simulink library "EarthAndTargetPointing"  (R2014b)
settings: Solver=ode45  StartTime=0.0  StopTime=10.0  RelTol=1e-3
undefined symbols (not defined in the file or in its folder): ConfParam
libraries: AdvancedMux x2, Normalization x2, AdvancedDemux x1, ComputeNorm3D x1, EarthPointing x1, ScalarProduct3D x1, TargetPointing x1
settings Model: Creator=Hp  LastModifiedBy=Hp

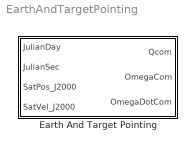
== system EarthAndTargetPointing ==
  Earth And Target Pointing : Subsystem

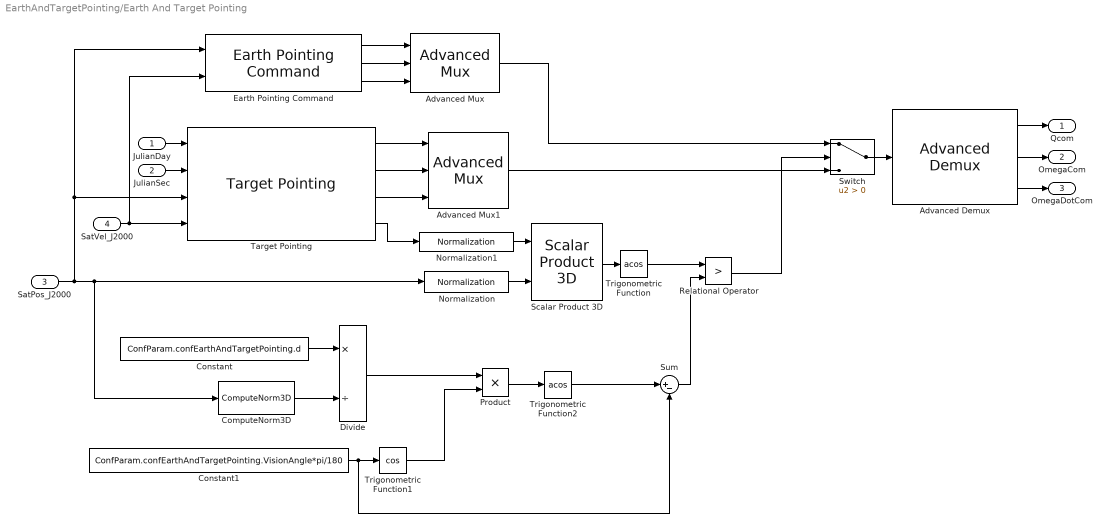
== system EarthAndTargetPointing/Earth And Target Pointing ==
  JulianDay : Inport
  JulianSec : Inport  Port=2
  SatPos_J2000 : Inport  Port=3
  SatVel_J2000 : Inport  Port=4
  Advanced Demux : AdvancedDemux/Advanced Demux
  Advanced Mux : AdvancedMux/Advanced Mux
  Advanced Mux1 : AdvancedMux/Advanced Mux
  ComputeNorm3D : ComputeNorm3D/ComputeNorm3D
  Constant : Constant  Value=ConfParam.confEarthAndTargetPointing.d
  Constant1 : Constant  Value=ConfParam.confEarthAndTargetPointing.VisionAngle*pi/180
  Divide : Product  Inputs=*/
  "Earth Pointing Command " : EarthPointing/Earth Pointing Command
  Normalization : Normalization/Normalization
  Normalization1 : Normalization/Normalization
  Product : Product
  Relational Operator : RelationalOperator  Operator=>  OutDataTypeStr=boolean
  Scalar Product 3D : ScalarProduct3D/Scalar Product 3D
  Sum : Sum  Inputs=|+-
  Switch : Switch  Criteria=u2 > Threshold
  Target Pointing : TargetPointing/Target Pointing
  Trigonometric Function : Trigonometry  Operator=acos
  Trigonometric Function1 : Trigonometry  Operator=cos
  Trigonometric Function2 : Trigonometry  Operator=acos
  Qcom : Outport
  OmegaCom : Outport  Port=2
  OmegaDotCom : Outport  Port=3
  wires:
  JulianSec/1 -> Target Pointing/2
  Normalization1/1 -> Scalar Product 3D/1
  Normalization/1 -> Scalar Product 3D/2
  SatPos_J2000/1 -> Target Pointing/3, "Earth Pointing Command "/1, ComputeNorm3D/1, Normalization/1
  JulianDay/1 -> Target Pointing/1
  Trigonometric Function/1 -> Relational Operator/1
  Scalar Product 3D/1 -> Trigonometric Function/1
  SatVel_J2000/1 -> Target Pointing/4, "Earth Pointing Command "/2
  Target Pointing/4 -> Normalization1/1
  "Earth Pointing Command "/1 -> Advanced Mux/1
  "Earth Pointing Command "/2 -> Advanced Mux/2
  "Earth Pointing Command "/3 -> Advanced Mux/3
  Target Pointing/1 -> Advanced Mux1/1
  Target Pointing/2 -> Advanced Mux1/2
  Target Pointing/3 -> Advanced Mux1/3
  Advanced Mux1/1 -> Switch/3
  Advanced Mux/1 -> Switch/1
  Switch/1 -> Advanced Demux/1
  Advanced Demux/1 -> Qcom/1
  Advanced Demux/2 -> OmegaCom/1
  Advanced Demux/3 -> OmegaDotCom/1
  Constant/1 -> Divide/1
  ComputeNorm3D/1 -> Divide/2
  Divide/1 -> Product/1
  Trigonometric Function1/1 -> Product/2
  Product/1 -> Trigonometric Function2/1
  Trigonometric Function2/1 -> Sum/1
  Constant1/1 -> Sum/2, Trigonometric Function1/1
  Sum/1 -> Relational Operator/2
  Relational Operator/1 -> Switch/2
